simulink model "NFO"  (R2023a)
settings: Solver=FixedStepDiscrete  StartTime=0.0  StopTime=10  FixedStep=TsModel  RelTol=1e-3
values from neighbouring files (symbols this model uses):
  ADRC_times = 1.0    [NFO.sldd]
  b0 = 10000.0    [NFO.sldd]
  CCR_Counter = 8000.0    [NFO.sldd]
  current_bandwidth = 1500.0    [NFO.sldd]
  FLL_K = 1.414    [NFO.sldd]
  flux = 0.011    [NFO.sldd]
  Idq_limit = 20.0    [NFO.sldd]
  IF_Initial = 40.0    [NFO.sldd]
  Ls = 0.0001952    [NFO.sldd]
  Min_FLL_omega = 10.0    [NFO.sldd]
  omega_c = 50.0    [NFO.sldd]
  PLL_I = 3000.0    [NFO.sldd]
  PLL_P = 10.0    [NFO.sldd]
  PMSM_B = 0.0004924    [NFO.sldd]
  PMSM_J = 0.0027    [NFO.sldd]
  PMSM_Pn = 5.0    [NFO.sldd]
  Pn = 5.0    [NFO.sldd]
  Rs = 0.1763    [NFO.sldd]
  Swich_time = 1.5    [NFO.sldd]
  tao = -30.0    [NFO.sldd]
  Ts = 0.0001    [NFO.sldd]
  TsModel = 2.5E-5    [NFO.sldd]
undefined symbols (not defined in the file or in its folder): DiscIntNeverNeededParam, sigbuilder_block
libraries: slpidlib x3, mcbplantlib x1, autolibpmsmexterior x1
(part 2 of 2)

== system NFO/Algorithm/IF_Gen/IFpos/integrator/RangeLimit ==
  In : Inport  OutDataTypeStr=single
  Constant : Constant  Value=2*pi  OutDataTypeStr=single  SampleTime=-1
  Constant1 : Constant  Value=0  OutDataTypeStr=single  SampleTime=-1
  If : If  NumInputs=2  IfExpression=u1  ElseIfExpressions=u2
  If Action Subsystem : Subsystem  TreatAsAtomicUnit=on
  If Action Subsystem1 : Subsystem  TreatAsAtomicUnit=on
  If Action Subsystem2 : Subsystem  TreatAsAtomicUnit=on
  Merge : Merge  Inputs=3
  Relational Operator : RelationalOperator  Operator=>  OutDataTypeStr=boolean  RndMeth=Simplest  InputSameDT=off
  Relational Operator1 : RelationalOperator  Operator=<  OutDataTypeStr=boolean  RndMeth=Simplest  InputSameDT=off
  Theta : Outport  OutDataTypeStr=single
  wires:
  Relational Operator/1 -> If/1
  Constant/1 -> Relational Operator/2
  Constant1/1 -> Relational Operator1/2
  In/1 -> Relational Operator1/1, If Action Subsystem2/1(In1), If Action Subsystem1/1(In1), If Action Subsystem/1(In1), Relational Operator/1
  Relational Operator1/1 -> If/2
  Merge/1 -> Theta/1
  If/3 -> If Action Subsystem2/Action
  If/2 -> If Action Subsystem/Action
  If/1 -> If Action Subsystem1/Action
  If Action Subsystem2/1(Out1) -> Merge/1
  If Action Subsystem/1(Out1) -> Merge/2
  If Action Subsystem1/1(Out1) -> Merge/3

== system NFO/Algorithm/SOSOIFO Obe/PLL/Inte_Limit/xianfu ==
  In : Inport  OutDataTypeStr=single
  Constant : Constant  Value=2*pi  OutDataTypeStr=single  SampleTime=-1
  Constant1 : Constant  Value=0  OutDataTypeStr=single  SampleTime=-1
  If : If  NumInputs=2  IfExpression=u1  ElseIfExpressions=u2
  If Action Subsystem : Subsystem  TreatAsAtomicUnit=on
  If Action Subsystem1 : Subsystem  TreatAsAtomicUnit=on
  If Action Subsystem2 : Subsystem  TreatAsAtomicUnit=on
  Merge : Merge  Inputs=3
  Relational Operator : RelationalOperator  Operator=>  OutDataTypeStr=boolean  RndMeth=Simplest  InputSameDT=off
  Relational Operator1 : RelationalOperator  Operator=<  OutDataTypeStr=boolean  RndMeth=Simplest  InputSameDT=off
  Theta : Outport  OutDataTypeStr=single
  wires:
  Relational Operator/1 -> If/1
  Constant/1 -> Relational Operator/2
  Constant1/1 -> Relational Operator1/2
  In/1 -> Relational Operator1/1, If Action Subsystem2/1(In1), If Action Subsystem1/1(In1), If Action Subsystem/1(In1), Relational Operator/1
  Relational Operator1/1 -> If/2
  Merge/1 -> Theta/1
  If/3 -> If Action Subsystem2/Action
  If/2 -> If Action Subsystem/Action
  If/1 -> If Action Subsystem1/Action
  If Action Subsystem2/1(Out1) -> Merge/1
  If Action Subsystem/1(Out1) -> Merge/2
  If Action Subsystem1/1(Out1) -> Merge/3

== system NFO/Algorithm/SOSOIFO Obe/SOSOIFO/SOSOGI_alpha/If Action Subsystem ==
  In1 : Inport  OutDataTypeStr=single
  Action Port : ActionPort  ActionPortLabel=else
  omega_e : Outport  OutDataTypeStr=single
  wires:
  In1/1 -> omega_e/1

== system NFO/Algorithm/SOSOIFO Obe/SOSOIFO/SOSOGI_alpha/If Action Subsystem2 ==
  In1 : Inport  OutDataTypeStr=single
  Action Port : ActionPort  ActionPortLabel=if(u1 < 0)
  omega_e : Outport  OutDataTypeStr=single
  wires:
  In1/1 -> omega_e/1

== system NFO/Algorithm/IF_Gen/IFneg/integrator/RangeLimit/If Action Subsystem ==
  In1 : Inport  OutDataTypeStr=single
  Action Port : ActionPort  ActionPortLabel=elseif(u2)
  Constant : Constant  Value=2*pi  OutDataTypeStr=single  SampleTime=-1
  Sum : Sum  Inputs=|++  OutDataTypeStr=single
  Out1 : Outport  OutDataTypeStr=single
  wires:
  Sum/1 -> Out1/1
  Constant/1 -> Sum/2
  In1/1 -> Sum/1

== system NFO/Algorithm/IF_Gen/IFneg/integrator/RangeLimit/If Action Subsystem1 ==
  In1 : Inport  OutDataTypeStr=single
  Action Port : ActionPort  ActionPortLabel=if(u1)
  Constant : Constant  Value=2*pi  OutDataTypeStr=single  SampleTime=-1
  Sum : Sum  Inputs=|+-  OutDataTypeStr=single
  Out1 : Outport  OutDataTypeStr=single
  wires:
  Sum/1 -> Out1/1
  Constant/1 -> Sum/2
  In1/1 -> Sum/1

== system NFO/Algorithm/IF_Gen/IFneg/integrator/RangeLimit/If Action Subsystem2 ==
  In1 : Inport  OutDataTypeStr=single
  Action Port : ActionPort  ActionPortLabel=else
  Out1 : Outport  OutDataTypeStr=single
  wires:
  In1/1 -> Out1/1

== system NFO/Algorithm/IF_Gen/IFpos/integrator/RangeLimit/If Action Subsystem ==
  In1 : Inport  OutDataTypeStr=single
  Action Port : ActionPort  ActionPortLabel=elseif(u2)
  Constant : Constant  Value=2*pi  OutDataTypeStr=single  SampleTime=-1
  Sum : Sum  Inputs=|++  OutDataTypeStr=single
  Out1 : Outport  OutDataTypeStr=single
  wires:
  In1/1 -> Sum/1
  Constant/1 -> Sum/2
  Sum/1 -> Out1/1

== system NFO/Algorithm/IF_Gen/IFpos/integrator/RangeLimit/If Action Subsystem1 ==
  In1 : Inport  OutDataTypeStr=single
  Action Port : ActionPort  ActionPortLabel=if(u1)
  Constant : Constant  Value=2*pi  OutDataTypeStr=single  SampleTime=-1
  Sum : Sum  Inputs=|+-  OutDataTypeStr=single
  Out1 : Outport  OutDataTypeStr=single
  wires:
  In1/1 -> Sum/1
  Constant/1 -> Sum/2
  Sum/1 -> Out1/1

== system NFO/Algorithm/IF_Gen/IFpos/integrator/RangeLimit/If Action Subsystem2 ==
  In1 : Inport  OutDataTypeStr=single
  Action Port : ActionPort  ActionPortLabel=else
  Out1 : Outport  OutDataTypeStr=single
  wires:
  In1/1 -> Out1/1

== system NFO/Algorithm/SOSOIFO Obe/PLL/Inte_Limit/xianfu/If Action Subsystem ==
  In1 : Inport  OutDataTypeStr=single
  Action Port : ActionPort  ActionPortLabel=elseif(u2)
  Constant : Constant  Value=2*pi  OutDataTypeStr=single  SampleTime=-1
  Sum : Sum  Inputs=|++  OutDataTypeStr=single
  Out1 : Outport  OutDataTypeStr=single
  wires:
  In1/1 -> Sum/1
  Constant/1 -> Sum/2
  Sum/1 -> Out1/1

== system NFO/Algorithm/SOSOIFO Obe/PLL/Inte_Limit/xianfu/If Action Subsystem1 ==
  In1 : Inport  OutDataTypeStr=single
  Action Port : ActionPort  ActionPortLabel=if(u1)
  Constant : Constant  Value=2*pi  OutDataTypeStr=single  SampleTime=-1
  Sum : Sum  Inputs=|+-  OutDataTypeStr=single
  Out1 : Outport  OutDataTypeStr=single
  wires:
  In1/1 -> Sum/1
  Constant/1 -> Sum/2
  Sum/1 -> Out1/1

== system NFO/Algorithm/SOSOIFO Obe/PLL/Inte_Limit/xianfu/If Action Subsystem2 ==
  In1 : Inport  OutDataTypeStr=single
  Action Port : ActionPort  ActionPortLabel=else
  Out1 : Outport  OutDataTypeStr=single
  wires:
  In1/1 -> Out1/1

== matlab function NFO/Algorithm/IF_Theta_Switch ==
  data: Time input; sensorless_theta output; IF_theta input; Obe_theta input; one input; zero input; theta_compa output; flag_1 output; Switch_time input
function [sensorless_theta,theta_compa,flag_1] = fcn(Time,IF_theta,Obe_theta,one,zero,Switch_time)
sensorless_theta=zero;
theta_compa=zero;
flag_1=zero;

%这里就是定义变量
persistent theta_give theta_comp last_error last_comp flag
if isempty(theta_give)
theta_give=zero+0.2;
theta_comp=zero;
last_error =one;
last_comp =zero;
flag=zero;
end

if(flag==1)
sensorless_theta =Obe_theta;
end


if(Time < Switch_time && flag==0 )
    sensorless_theta=  IF_theta; %当前面一个模块的输出的计数时间小于我们的IF切换时间，这里是1.5s,这里用的是IF的角度
elseif(Switch_time <=Time && Time <=Switch_time+0.05 && flag==0) %0.05秒内完成切换
    %当运行时间大于切换角度，并且小于切换时间+0.05s，这里表示要在0.05内完成切换
   % theta_comp = 1.0e-04 * 0.999950001666625*last_error + 0.999900004999833*last_comp ;  
    theta_comp =  0.009950166250832*last_error + 0.990049833749168*last_comp ;  
    %0.01Tc
    theta_compa = theta_comp;
    theta_give = IF_theta + theta_comp;
    sensorless_theta = theta_give; %这是使用的角度
    if( sensorless_theta- Obe_theta<0.1 && sensorless_theta- Obe_theta>-0.1)
        flag=one; %当我们使用的角度和观测器输出的角度很小，小于0.1,可以认为此时已经切换成功了
    end
end
last_error = (Obe_theta-IF_theta);
last_comp= theta_comp;
if(sensorless_theta- Obe_theta<0.2 && sensorless_theta- Obe_theta>-0.2)
    flag_1=one;
end

== matlab function NFO/Algorithm/IF_Current_Switch ==
  data: Time input; Iq output; IF_iq input; Speed_iq input; Cos_error input; Swich_time input
function Iq  = fcn(Time,IF_iq,Speed_iq,Cos_error,Swich_time)
Iq=IF_iq;
persistent real_Iq last_iq IF_q
if isempty(real_Iq)
real_Iq=Cos_error;
last_iq=Iq;
IF_q=Iq;
end

%电流环节是递减的过程
if(Time < Swich_time)
    Iq=  IF_iq;
    real_Iq=Cos_error;
elseif( Swich_time<= Time && Time <= Swich_time+0.05)
%    Iq=   1.0e-04 *0.612481242570466*real_Iq + 0.999938751875743*last_iq; %  0.01/6.125Tc
   Iq=  0.059411936635658*real_Iq + 0.940588063364342*last_iq; %  0.01/6.125Tc
% elseif( 3.5 <= Time && Time <= 4.5)
%     if(Speed_iq<IF_q)
%         Iq=IF_q;
%     else
%         Iq= Speed_iq;
%     end
else
    Iq= Speed_iq;
end
init=real_Iq;
last_iq=Iq;

== matlab function NFO/Algorithm/IF_theta_Select ==
  data: input input; IF_theta output; pos_theta input; pos_omega input; neg_theta input; neg_omega input; IF_omega output
function [IF_theta,IF_omega] = fcn(input,pos_theta,pos_omega,neg_theta,neg_omega)
if(input == 0)
IF_theta = neg_theta;
IF_omega=neg_omega;
else
IF_theta=  pos_theta;
IF_omega=pos_omega;
end

== matlab function NFO/Algorithm/ Switch_Counter ==
  data: flag_Set_dir_0neg_1pos output single; T_omega input single; one input single; zero input single; time_count output single; omega_T output single
function [flag_Set_dir_0neg_1pos, time_count,omega_T] = fcn(T_omega,one,zero)
time_count=zero;   %计时时间仿真看
flag_Set_dir_0neg_1pos=zero;%IF启动方向选择
omega_T=T_omega;    %给定角速度
persistent time%time也为计时时间
if isempty(time)
time=zero;
end

%判断目标速度的正负
if(T_omega>30)
flag_Set_dir_0neg_1pos = one;
   time = time + 0.0001;%离散积分，算法运行频率10khz，time_count为IF启动运行时间
   time_count=time;
elseif(T_omega<-30)
flag_Set_dir_0neg_1pos = zero;
   time = time + 0.0001;%离散积分，算法运行频率10khz，time_count为IF启动运行时间
   time_count=time;
end
end
